simulink model "ysw5_15"  (R2014a)
settings: Solver=ode45  StartTime=0.0  StopTime=10.0  RelTol=1e-3
settings Model: Creator=Administrator  LastModifiedBy=Administrator

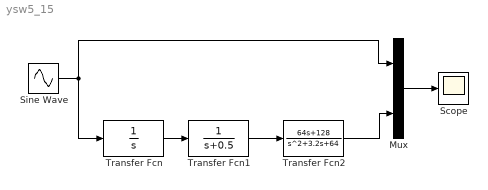
== system ysw5_15 ==
  Mux : Mux  Inputs=2
  Scope : Scope
  Sine Wave : Sin  SampleTime=0
  Transfer Fcn : TransferFcn  Denominator=[1 0]
  Transfer Fcn1 : TransferFcn  Denominator=[1 0.5]
  Transfer Fcn2 : TransferFcn  Numerator=[64 128]  Denominator=[1 3.2 64]
  wires:
  Sine Wave/1 -> Mux/1, Transfer Fcn/1
  Transfer Fcn1/1 -> Transfer Fcn2/1
  Transfer Fcn/1 -> Transfer Fcn1/1
  Mux/1 -> Scope/1
  Transfer Fcn2/1 -> Mux/2
